simulink model "MPC2"  (R2021b)
settings: Solver=VariableStepAuto  StartTime=0.0  StopTime=200  RelTol=1e-3
values from neighbouring files (symbols this model uses):
  A1 = [0 0 1 0 ; 0 0 0 1 ; 0 A132 A133 A134 ; 0 A142 A143 A144]    [NXTway_model.m]    (also in SS_matrices.m)
  B1 = [0 0 ; 0 0 ; B13 B13 ; B14 B14]    [NXTway_model.m]    (also in SS_matrices.m)
  C1 = [1 0 0 0 ; 0 1 0 0]    [SS_matrices.m]
  D1 = [0 0 ; 0 0]    [SS_matrices.m]
undefined symbols (not defined in the file or in its folder): Continuous, Time
libraries: simulink x1, ctrlSharedLib x1, mpclib x1
settings Model: Creator=oliverschamp  LastModifiedBy=oliverschamp

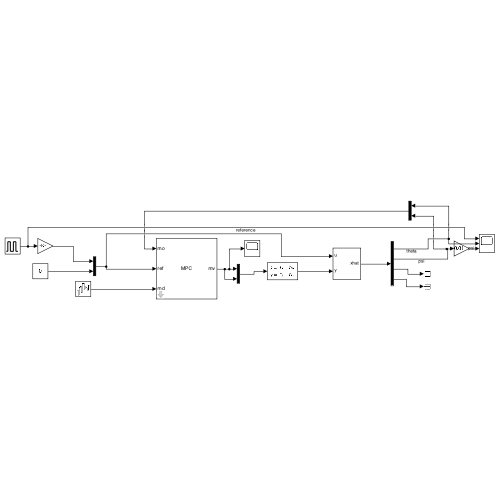
[thumbnail: Simulink's stored preview of the top-level diagram]
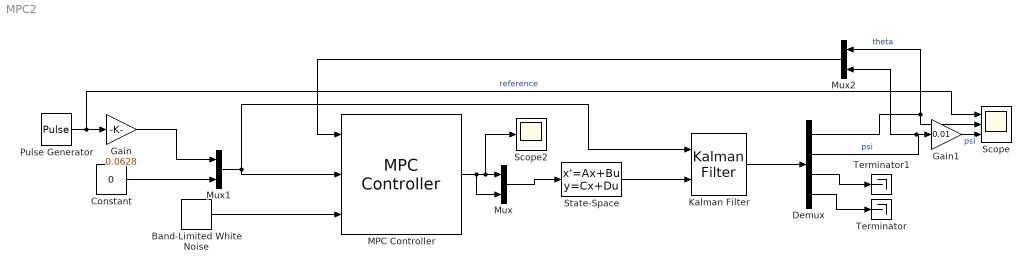
== system MPC2 ==
  Band-Limited White Noise : simulink/Sources/Band-Limited White Noise  Cov=[0]  Ts=0.1  seed=[23341]
  Constant : Constant  Value=0
  Demux : Demux
  Gain : Gain  Gain=0.0628
  Gain1 : Gain  Gain=0.01
  Kalman Filter : ctrlSharedLib/Kalman Filter  TimeDomain=Continuous-Time  UseCurrentEstimator=on  ModelSource=LTI State-Space Variable  ModelSourceVariable=sys1  A=0.95  B=1  C=1  D=0  NumberOfStates=1  NumberOfInputs=1  NumberOfOutputs=1  InitialEstimateSource=Dialog  X0=[0 0 0 0]  P0=10  UseK=off  UseGH=off  NumberOfProcessNoiseInputs=1  G=1  TimeInvariantG=on  H=0  TimeInvariantH=on  Q=0.05  TimeInvariantQ=on  R=1  TimeInvariantR=on  N=0  TimeInvariantN=on  AddInputPort=on  AddEnablePort=off  OutputEstimatedY=off  OutputP=off  Ts=-1
  MPC Controller : mpclib/MPC Controller  SCDEnableBlockLinearizationSpecification=on  mpcobj=mpc1  is_multiple=0  enable_value=0  return_u0=off  updateMPCinCallerWorkspace=on  md_inport=on  mv_inport=off  uref_inport=off  return_cost=off  return_mvseq=off  return_qpstatus=off  return_xseq=off  return_state=off  return_ovseq=off  state_inport=off  umin_inport=off  umax_inport=off  ymin_inport=off  ymax_inport=off  cc_inport=off  ywt_inport=off  uwt_inport=off  duwt_inport=off  rhoeps_inport=off  pm_inport=off  MaximumP=10  HorizonChoice=FixedHorizon  n_ts=0.1  n_p=15  n_mv=1  n_md=1  n_ud=0  n_mo=2  n_uo=0  BlockDataType=double  SampleTimeInherited=off  switch_inport=off
  Mux : Mux  Inputs=2
  Mux1 : Mux  Inputs=2
  Mux2 : Mux  Inputs=2
  Pulse Generator : DiscretePulseGenerator  PulseType=Time based  Amplitude=20  Period=100  PulseWidth=50
  Scope : Scope  NumInputPorts=3
  Scope2 : Scope
  State-Space : StateSpace  A=A1  B=B1  C=C1  D=D1  InitialCondition=[0 0 0 0]
  Terminator : Terminator
  Terminator1 : Terminator
  wires:
  Constant/1 -> Mux1/2
  MPC Controller/1 -> Mux/2, Scope2/1, Mux/1
  Demux/1 -> Mux2/1, Scope/2  "theta"
  Pulse Generator/1 -> Scope/1, Gain/1  "reference"
  Mux2/1 -> MPC Controller/1
  Gain/1 -> Mux1/1
  Demux/4 -> Terminator/1
  Mux/1 -> State-Space/1
  Demux/3 -> Terminator1/1
  Kalman Filter/1 -> Demux/1
  Mux1/1 -> MPC Controller/2, Kalman Filter/1
  State-Space/1 -> Kalman Filter/2
  Demux/2 -> Gain1/1, Mux2/2  "psi"
  Gain1/1 -> Scope/3  "psi"
  Band-Limited White Noise/1 -> MPC Controller/3
